simulink model "ammclib_amclib_current_loop_s32k14x"  (Simulink 9.0)
settings: Solver=FixedStepDiscrete  StartTime=0.0  StopTime=10  FixedStep=0.001  RelTol=1e-3  EnableMultiTasking=on
InitFcn:
  | mbd_s32k_consistency_checks(bdroot(gcs));
undefined symbols (not defined in the file or in its folder): LQFP
libraries: ammclib_bam_s32k14x x11, simulink x7, mbd_s32k1xx_ec_toolbox x2
Description:
  | This model tests the AMMCLIB AMCLIB Current Loop blocks
  | 
  | Validation:
  | - Run the model in Simulation and compare the Inputs vs Outputs results.
  | - Open Freemaster (ammclib_amclib_current_loop_s32k14x.pmp) and compare the HW results against the Simulated ones
settings Model: Creator=NXP MBDT Team  LastModifiedBy=nxf35172
settings DataIOCC: ExternalInput=off  InitialState=off  LimitDataPoints=on  SaveOutput=off  SignalLogging=off  SaveTime=off
settings OptimizationCC: DefaultParameterBehavior=Inlined  LifeSpan=1
settings DebuggingCC: SolverPrmCheckMsg=warning  InheritedTsInSrcMsg=none  SingleTaskRateTransMsg=error  ParameterPrecisionLossMsg=none  UnconnectedInputMsg=error  UnconnectedOutputMsg=error  UnconnectedLineMsg=error  AllowSymbolicDim=off  UnknownTsInhSupMsg=error  StateNameClashWarn=warning
settings HardwareCC: ProdLargestAtomicInteger=Long  ProdLargestAtomicFloat=Double  ProdEndianess=LittleEndian  ProdHWDeviceType=ARM Compatible->ARM Cortex
settings SFSimCC: MATLABDynamicMemAlloc=off
settings RTWCC: SystemTargetFile=mbd_s32k.tlc  MakeCommand=mbd_s32k_make_rtw COPY_MDLREF_INCLUDES=0  TemplateMakefile=mbd_s32k.tmf  Description=Model Based Design Toolbox S32K14x Code Generation Target
settings CodeAppCC: IgnoreCustomStorageClasses=off
settings STFCustomTargetCC: CombineOutputUpdateFcns=on  ERTCustomFileBanners=on  SupportContinuousTime=off  SupportNonInlinedSFcns=off  RemoveResetFunc=on  MATLABClassNameForMDSCustomization=Simulink.SoftwareTarget.ERTCustomization  GRTInterface=off  SystemTargetFile=mbd_s32k14.tlc
settings ERTTargetCC: MultiwordLength=2048  ParMdlRefBuildCompliant=off  CompOptLevelCompliant=off  ConcurrentExecutionCompliant=off  ModelStepFunctionPrototypeControlCompliant=off  CPPClassGenCompliant=off  UseToolchainInfoCompliant=off  InlinedParameterPlacement=NonHierarchical  ERTCustomFileTemplate=example_file_process.tlc  ConvertIfToSwitch=off  SuppressUnreachableDefaultCases=off

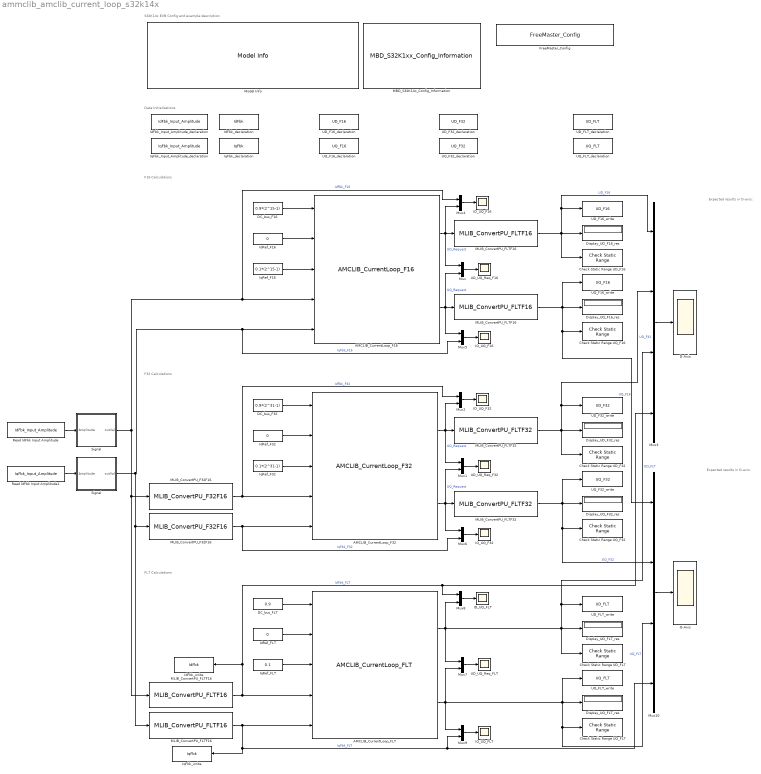
== system ammclib_amclib_current_loop_s32k14x ==
  note: Expected results in D-axis:
  note: S32K14x EVB Config and example description
  note: Data Initializations
  note: F16 Calculations
  note: F32 Calculations
  note: FLT Calculations
  note: Expected results in D-axis:
  " MLIB_ConvertPU_FLTF16   " : ammclib_bam_s32k14x/MLIB/bam_flt/MLIB_ConvertPU_FLTF16
  AMCLIB_CurrentLoop_F16 : ammclib_bam_s32k14x/AMCLIB/bam_f16/AMCLIB_CurrentLoop_F16  f16CC1scD=0.006*(2^15-1)  f16CC2scD=0.006*(2^15-1)  u16NShiftD=0  f16CC1scQ=0.006*(2^15-1)  f16CC2scQ=0.006*(2^15-1)  u16NShiftQ=0
  AMCLIB_CurrentLoop_F32 : ammclib_bam_s32k14x/AMCLIB/bam_f32/AMCLIB_CurrentLoop_F32  f32CC1scD=0.006*(2^31-1)  f32CC2scD=0.006*(2^31-1)  u16NShiftD=0  f32CC1scQ=0.006*(2^31-1)  f32CC2scQ=0.006*(2^31-1)  u16NShiftQ=0
  AMCLIB_CurrentLoop_FLT : ammclib_bam_s32k14x/AMCLIB/bam_flt/AMCLIB_CurrentLoop_FLT  fltCC1scD=0.006  fltCC2scD=0.006  fltCC1scQ=0.006  fltCC2scQ=0.006
  Check Static Range UD_F16 : simulink/Model Verification/Check  Static Range  Description=-0.9*(2^15-1) <= u <= 0.9*(2^15-1)  max=0.9*(2^15-1)  max_included=on  min=-0.9*(2^15-1)  min_included=on  enabled=on  stopWhenAssertionFail=on  export=off  icon=graphic
      settings: SourceProductName=Simulink  SourceProductBaseCode=SL
  Check Static Range UD_F32 : simulink/Model Verification/Check  Static Range  Description=-0.9*(2^31-1) <= u <= 0.9*(2^31-1)  max=0.9*(2^31-1)  max_included=on  min=-0.9*(2^31-1)  min_included=on  enabled=on  stopWhenAssertionFail=on  export=off  icon=graphic
      settings: SourceProductName=Simulink  SourceProductBaseCode=SL
  Check Static Range UD_FLT : simulink/Model Verification/Check  Static Range  Description=-0.9 <= u <= 0.9  max=0.9  max_included=on  min=-0.9  min_included=on  enabled=on  stopWhenAssertionFail=on  export=off  icon=graphic
      settings: SourceProductName=Simulink  SourceProductBaseCode=SL
  "Check Static Range UQ_F16 " : simulink/Model Verification/Check  Static Range  Description=-0.9*(2^15-1) <= u <= 0.9*(2^15-1)  max=0.9*(2^15-1)  max_included=on  min=-0.9*(2^15-1)  min_included=on  enabled=on  stopWhenAssertionFail=on  export=off  icon=graphic
      settings: SourceProductName=Simulink  SourceProductBaseCode=SL
  Check Static Range UQ_F32 : simulink/Model Verification/Check  Static Range  Description=-0.9*(2^31-1) <= u <= 0.9*(2^31-1)  max=0.9*(2^31-1)  max_included=on  min=-0.9*(2^31-1)  min_included=on  enabled=on  stopWhenAssertionFail=on  export=off  icon=graphic
      settings: SourceProductName=Simulink  SourceProductBaseCode=SL
  Check Static Range UQ_FLT : simulink/Model Verification/Check  Static Range  Description=-0.9 <= u <= 0.9  max=0.9  max_included=on  min=-0.9  min_included=on  enabled=on  stopWhenAssertionFail=on  export=off  icon=graphic
      settings: SourceProductName=Simulink  SourceProductBaseCode=SL
  D-Axis : Scope
  DC_bus_F16 : Constant  Value=0.9*(2^15-1)  OutDataTypeStr=Inherit: Inherit via back propagation
  DC_bus_F32 : Constant  Value=0.9*(2^31-1)  OutDataTypeStr=Inherit: Inherit via back propagation
  DC_bus_FLT : Constant  Value=0.9  OutDataTypeStr=Inherit: Inherit via back propagation
  Display_UD_F16_res : Display
  Display_UD_F32_res : Display
  Display_UD_FLT_res : Display
  Display_UQ_F16_res : Display
  Display_UQ_F32_res : Display
  Display_UQ_FLT_res : Display
  FreeMaster_Config : mbd_s32k1xx_ec_toolbox/Utility Blocks/FreeMaster_Config  interface=LPUART1  baudrate=115200  rxd=PTC6: [LPUART1_RX | Receive]  txd=PTC7: [LPUART1_TX | Transmit]  mode=Short Interrupt  isr_prio=1  show_adv_opts=on  use_scope=on  max_scope_vars=8  use_recorder=on  max_rec_vars=8  rec_buff_size=1024  rec_timebase=0 milliseconds  comm_buffer_size_auto=on  comm_buffer_size=255  comm_rqueue_size_default=on  comm_rqueue_size=32
  ID_UQ_F16 : Scope
  ID_UQ_F32 : Scope
  ID_UQ_FLT : Scope
  IQ_UQ_F16 : Scope
  IQ_UQ_F32 : Scope
  IQ_UQ_FLT : Scope
  IdFbk_Input_Amplitude_declaration : DataStoreMemory  Priority=1  DataStoreName=IdFbk_Input_Amplitude  WriteAfterWriteMsg=warning  WriteAfterReadMsg=warning  InitialValue=0.25*(2^15-1)  ShowAdditionalParam=off  OutMin=-32768  OutMax=32767  OutDataTypeStr=int16
  IdFbk_declaration : DataStoreMemory  Priority=1  DataStoreName=IdFbk  WriteAfterWriteMsg=warning  WriteAfterReadMsg=warning  ShowAdditionalParam=off  OutMin=-1  OutMax=1  OutDataTypeStr=single
  IdFbk_write : DataStoreWrite  DataStoreName=IdFbk
  IdRef_F16 : Constant  Value=0  OutDataTypeStr=Inherit: Inherit via back propagation
  IdRef_F32 : Constant  Value=0  OutDataTypeStr=Inherit: Inherit via back propagation
  IdRef_FLT : Constant  Value=0  OutDataTypeStr=Inherit: Inherit via back propagation
  IqFbk_Input_Amplitude_declaration : DataStoreMemory  Priority=1  DataStoreName=IqFbk_Input_Amplitude  WriteAfterWriteMsg=warning  WriteAfterReadMsg=warning  InitialValue=0.25*(2^15-1)  ShowAdditionalParam=off  OutMin=-32768  OutMax=32767  OutDataTypeStr=int16
  IqFbk_declaration : DataStoreMemory  Priority=1  DataStoreName=IqFbk  WriteAfterWriteMsg=warning  WriteAfterReadMsg=warning  ShowAdditionalParam=off  OutMin=-1  OutMax=1  OutDataTypeStr=single
  IqFbk_write : DataStoreWrite  DataStoreName=IqFbk
  IqRef_F16 : Constant  Value=0.1*(2^15-1)  OutDataTypeStr=Inherit: Inherit via back propagation
  IqRef_F32 : Constant  Value=0.1*(2^31-1)  OutDataTypeStr=Inherit: Inherit via back propagation
  IqRef_FLT : Constant  Value=0.1  OutDataTypeStr=Inherit: Inherit via back propagation
  MBD_S32K14x_Config_Information : mbd_s32k1xx_ec_toolbox/MBD_S32K1xx_Config_Information  Priority=0  mbdt_ver=0  disp_str=|  config_params=[]  mcu_target_name=S32K144  mcu_target_package=100-LQFP  mcu_target_sram_size=64KB  mcu_system_clock_freq=80  mcu_xtal_freq=External 8  mcu_steptick_timer=LPIT Channel 0  mcu_steptick_prio=15  ds_import_enable=on  target_compiler=GCC  target_memory=FLASH  gcc_target_compile_opts=-mcpu=cortex-m4 -mthumb -mfloat-abi=hard -mfpu=fpv4-sp-d16 -O1 -g -gstrict-dwarf  gcc_target_assemble_opts=-mcpu=cortex-m4 -mthumb -mfloat-abi=hard -mfpu=fpv4-sp-d16 -g  gcc_target_link_opts=-mcpu=cortex-m4 -mthumb -mfloat-abi=hard -mfpu=fpv4-sp-d16  gcc_target_default_lcf=on  gcc_target_user_lcf=S32K144_64_flash.ld  ghs_target_compile_opts=-cpu=cortexm4f -thumb -DARM_MATH_CM4 -fpu=vfpv4_d16 -fsingle -Ogeneral -Wundef -Wimplicit-int -Wshadow -Wtrigraphs --no_commons --gnu_asm -gnu99 -gdwarf-2 -G  ghs_target_assemble_opts=-cpu=cortexm4f -fpu=vfpv4_d16  ghs_target_link_opts=-cpu=cortexm4f -thumb -fpu=vfpv4_d16  ghs_target_default_lcf=off  ghs_target_user_lcf=S32K144_64_flash.ld  iar_target_compile_opts=--cpu=Cortex-M4F --thumb --fpu=VFPv4_sp -Ol -e --debug --dlib_config normal  iar_target_assemble_opts=--cpu Cortex-M4F --thumb --fpu VFPv4_sp  iar_target_link_opts=--no_exceptions --vfe --inline  iar_target_default_lcf=off  iar_target_user_lcf=S32K144_64_flash.icf  pil_download_enable=off  rbl_download_enable=on  rbl_start_delay=5000000  rbl_download_interface=OpenSDA  rbl_restart_request=off  rbl_com_port=Custom  rbl_com_port_custom=COM1  pil_download_rate=57600  pil_opensda_drive=Custom  pil_opensda_drive_custom=D  pil_uart_instance=0  pil_uart_rx=PTA2: [LPUART0_RX | Receive]  pil_uart_tx=PTA3: [LPUART0_TX | Transmit]  FTM_PWM_PcrCheckEnDis=on  FTM_Input_Edge_Inputs_PcrCheckEnDis=on  FTM_Dual_Edge_Inputs_PcrCheckEnDis=on  FTM_Quadrature_Inputs_PcrCheckEnDis=on  FTM_Hall_Sensor_Inputs_PcrCheckEnDis=on  LPTMR_PcrCheckEnDis=on  PIT_PcrCheckEnDis=on  RTC_PcrCheckEnDis=on  FlexCAN_PcrCheckEnDis=on  LIN_PcrCheckEnDis=on  FlexIO_PcrCheckEnDis=on  LPI2C_PcrCheckEnDis=on  LPSPI_PcrCheckEnDis=on  LPUART_PcrCheckEnDis=on  CMP_PcrCheckEnDis=on  GPIO_OutputPcrCheckEnDis=on  GPIO_InputPcrCheckEnDis=on  SBC_PcrCheckEnDis=on  AMMCLIB_PcrCheckEnDis=on  FM_PcrCheckEnDis=on  Profile_PcrCheckEnDis=on  ConfigParams_PcrCheckEnDis=on  ModelRef_PcrCheckEnDis=on  PDB0_PcrCheckEnDis=on  CSEc_PcrCheckEnDis=on  eDMA_PcrCheckEnDis=on  ADC_PcrCheckEnDis=on  WDOG_PcrCheckEnDis=on
      | Target : S32K142-16KB_SRAM
      | Package : 100-pin
      | System clock : 80 MHz
      | XTAL clock : External 8 MHz
      | Compiler : GCC
      | Target Type : FLASH
      | Download Code after build : (OpenSDA: E)
      | Step Tick Interrupt Priority : 15
  "MLIB_ConvertPU_F32F16 " : ammclib_bam_s32k14x/MLIB/bam_f32/MLIB_ConvertPU_F32F16
  "MLIB_ConvertPU_F32F16  " : ammclib_bam_s32k14x/MLIB/bam_f32/MLIB_ConvertPU_F32F16
  "MLIB_ConvertPU_FLTF16  " : ammclib_bam_s32k14x/MLIB/bam_flt/MLIB_ConvertPU_FLTF16
  "MLIB_ConvertPU_FLTF16   " : ammclib_bam_s32k14x/MLIB/bam_flt/MLIB_ConvertPU_FLTF16
  "MLIB_ConvertPU_FLTF16    " : ammclib_bam_s32k14x/MLIB/bam_flt/MLIB_ConvertPU_FLTF16
  MLIB_ConvertPU_FLTF32 : ammclib_bam_s32k14x/MLIB/bam_flt/MLIB_ConvertPU_FLTF32
  "MLIB_ConvertPU_FLTF32  " : ammclib_bam_s32k14x/MLIB/bam_flt/MLIB_ConvertPU_FLTF32
  Model Info : simulink/Model-Wide Utilities/Model Info  Frame=off  DisplayStringWithTags=|  HorizontalTextAlignment=Left  LeftAlignmentValue=0.02
      | Model Name: %<ModelName>
      | 
      | Description: %<Description>
  Mux{,1..2,4..9} (9 alike) : Mux  Inputs=2
  Mux10 : Mux
  Mux3 : Mux
  Q-Axis : Scope
  Read IdFbk Input Amplitude : DataStoreRead  DataStoreName=IdFbk_Input_Amplitude
  Read IdFbk Input Amplitude1 : DataStoreRead  DataStoreName=IqFbk_Input_Amplitude
  Signal : Stateflow chart  TreatAsAtomicUnit=on
  "Signal " : Stateflow chart  TreatAsAtomicUnit=on
  UD_F16_declaration : DataStoreMemory  Priority=2  DataStoreName=UD_F16  ReadBeforeWriteMsg=warning  WriteAfterWriteMsg=warning  WriteAfterReadMsg=warning  ShowAdditionalParam=off  OutDataTypeStr=single
  UD_F16_write : DataStoreWrite  DataStoreName=UD_F16
  UD_F32_declaration : DataStoreMemory  Priority=2  DataStoreName=UD_F32  ReadBeforeWriteMsg=warning  WriteAfterWriteMsg=warning  WriteAfterReadMsg=warning  ShowAdditionalParam=off  OutDataTypeStr=single
  UD_F32_write : DataStoreWrite  DataStoreName=UD_F32
  UD_FLT_declaration : DataStoreMemory  Priority=2  DataStoreName=UD_FLT  ReadBeforeWriteMsg=warning  WriteAfterWriteMsg=warning  WriteAfterReadMsg=warning  ShowAdditionalParam=off  OutDataTypeStr=single
  UD_FLT_write : DataStoreWrite  DataStoreName=UD_FLT
  UD_UQ_Req_F16 : Scope
  UD_UQ_Req_F32 : Scope
  UD_UQ_Req_FLT : Scope
  UQ_F16_declaration : DataStoreMemory  Priority=3  DataStoreName=UQ_F16  ReadBeforeWriteMsg=warning  WriteAfterWriteMsg=warning  WriteAfterReadMsg=warning  ShowAdditionalParam=off  OutDataTypeStr=single
  UQ_F16_write : DataStoreWrite  DataStoreName=UQ_F16
  UQ_F32_declaration : DataStoreMemory  Priority=3  DataStoreName=UQ_F32  ReadBeforeWriteMsg=warning  WriteAfterWriteMsg=warning  WriteAfterReadMsg=warning  ShowAdditionalParam=off  OutDataTypeStr=single
  UQ_F32_write : DataStoreWrite  DataStoreName=UQ_F32
  UQ_FLT_declaration : DataStoreMemory  Priority=3  DataStoreName=UQ_FLT  ReadBeforeWriteMsg=warning  WriteAfterWriteMsg=warning  WriteAfterReadMsg=warning  ShowAdditionalParam=off  OutDataTypeStr=single
  UQ_FLT_write : DataStoreWrite  DataStoreName=UQ_FLT
  wires:
  Read IdFbk Input Amplitude/1 -> Signal/1(Amplitude)
  DC_bus_F16/1 -> AMCLIB_CurrentLoop_F16/1
  AMCLIB_CurrentLoop_F16/2 -> Mux5/1, Mux/2, "MLIB_ConvertPU_FLTF16   "/1  "UQ_Request"
  "MLIB_ConvertPU_FLTF16   "/1 -> Mux10/1, "Check Static Range UQ_F16 "/1, UQ_F16_write/1, Display_UQ_F16_res/1  "UQ_F16"
  Mux3/1 -> D-Axis/1
  AMCLIB_CurrentLoop_F16/1 -> Mux4/2, Mux/1, " MLIB_ConvertPU_FLTF16   "/1  "UD_Request"
  " MLIB_ConvertPU_FLTF16   "/1 -> Check Static Range UD_F16/1, Mux3/1, UD_F16_write/1, Display_UD_F16_res/1  "UD_F16"
  IdRef_F16/1 -> AMCLIB_CurrentLoop_F16/2
  IqRef_F16/1 -> AMCLIB_CurrentLoop_F16/3
  Read IdFbk Input Amplitude1/1 -> "Signal "/1(Amplitude)
  Mux/1 -> UD_UQ_Req_F16/1
  Mux4/1 -> ID_UQ_F16/1
  Mux5/1 -> IQ_UQ_F16/1
  DC_bus_F32/1 -> AMCLIB_CurrentLoop_F32/1
  AMCLIB_CurrentLoop_F32/2 -> "MLIB_ConvertPU_FLTF32  "/1, Mux6/1, Mux1/2  "UQ_Request"
  "MLIB_ConvertPU_FLTF32  "/1 -> Mux10/2, Check Static Range UQ_F32/1, UQ_F32_write/1, Display_UQ_F32_res/1  "UQ_F32"
  AMCLIB_CurrentLoop_F32/1 -> MLIB_ConvertPU_FLTF32/1, Mux2/2, Mux1/1  "UD_Request"
  MLIB_ConvertPU_FLTF32/1 -> Check Static Range UD_F32/1, Mux3/2, UD_F32_write/1, Display_UD_F32_res/1  "UD_F32"
  IdRef_F32/1 -> AMCLIB_CurrentLoop_F32/2
  IqRef_F32/1 -> AMCLIB_CurrentLoop_F32/3
  Mux1/1 -> UD_UQ_Req_F32/1
  Mux2/1 -> ID_UQ_F32/1
  Mux6/1 -> IQ_UQ_F32/1
  "MLIB_ConvertPU_F32F16 "/1 -> AMCLIB_CurrentLoop_F32/4, Mux2/1  "IdFbk_F32"
  "MLIB_ConvertPU_F32F16  "/1 -> AMCLIB_CurrentLoop_F32/5, Mux6/2  "IqFbk_F32"
  DC_bus_FLT/1 -> AMCLIB_CurrentLoop_FLT/1
  Signal/1(outVal) -> "MLIB_ConvertPU_FLTF16  "/1, "MLIB_ConvertPU_F32F16 "/1, Mux4/1, AMCLIB_CurrentLoop_F16/4  "IdFbk_F16"
  AMCLIB_CurrentLoop_FLT/1 -> Check Static Range UD_FLT/1, Mux3/3, UD_FLT_write/1, Display_UD_FLT_res/1, Mux8/2, Mux7/1  "UD_FLT"
  IdRef_FLT/1 -> AMCLIB_CurrentLoop_FLT/2
  IqRef_FLT/1 -> AMCLIB_CurrentLoop_FLT/3
  "Signal "/1(outVal) -> "MLIB_ConvertPU_FLTF16    "/1, "MLIB_ConvertPU_F32F16  "/1, Mux5/2, AMCLIB_CurrentLoop_F16/5  "IqFbk_F16"
  Mux7/1 -> UD_UQ_Req_FLT/1
  Mux8/1 -> ID_UQ_FLT/1
  Mux9/1 -> IQ_UQ_FLT/1
  "MLIB_ConvertPU_FLTF16  "/1 -> AMCLIB_CurrentLoop_FLT/4, IdFbk_write/1, Mux3/4, Mux8/1  "IdFbk_FLT"
  "MLIB_ConvertPU_FLTF16    "/1 -> AMCLIB_CurrentLoop_FLT/5, IqFbk_write/1, Mux10/4, Mux9/2  "IqFbk_FLT"
  AMCLIB_CurrentLoop_FLT/2 -> Mux10/3, Check Static Range UQ_FLT/1, UQ_FLT_write/1, Display_UQ_FLT_res/1, Mux9/1, Mux7/2  "UQ_FLT"
  Mux10/1 -> Q-Axis/1

== stateflow chart Signal ==
  settings: executeAtInitialization=1
  state A
    du:
    outVal = Amplitude;
    cntr=cntr+1;
  state A1
    du:
    outVal = -Amplitude;
    cntr=cntr-1;
  (default) -> A : {cntr=0;}
  A1 -> A : [cntr < 2]
  A -> A1 : [cntr > 1000]
  data: cntr local uint32 [0..12] =0; outVal output int16; Amplitude input int16

== stateflow chart Signal  ==
  settings: executeAtInitialization=1
  state A
    du:
    outVal = Amplitude;
    cntr=cntr+1;
  state A1
    du:
    outVal = -Amplitude;
    cntr=cntr-1;
  (default) -> A : {cntr=0;}
  A1 -> A : [cntr < 2]
  A -> A1 : [cntr > 1000]
  data: cntr local uint32 [0..12] =0; outVal output int16; Amplitude input int16
